simulink model "test_gFunction"  (R2018b)
settings: Solver=ode23  StartTime=0.0  StopTime=50*24*3600  RelTol=1e-3
values from neighbouring files (symbols this model uses):
  c4 = c41    [parameter_CARNOTews.m]
  gfunction = zeros(length(t_Trichter),length(r_Trichter))    [parameter_CARNOTews.m]
  L1 = 1/R1    [parameter_CARNOTews.m]
  lambdaErde = 2.0    (= 2)    [parameter_CARNOTews.m]
  Rechenradius = rm    (= 5)    [parameter_CARNOTews.m]
  T_null = TEarth0(end,:)'    [parameter_CARNOTews.m]
  t_start = 50*8560*3600    (= 1540800000)    [parameter_CARNOTews.m]
  Ts_Trichter = 7*24*3600    (= 604800)    [parameter_CARNOTews.m]
undefined symbols (not defined in the file or in its folder): dl
settings Model: SimulationMode=accelerator  Creator=drhf  LastModifiedBy=drhf

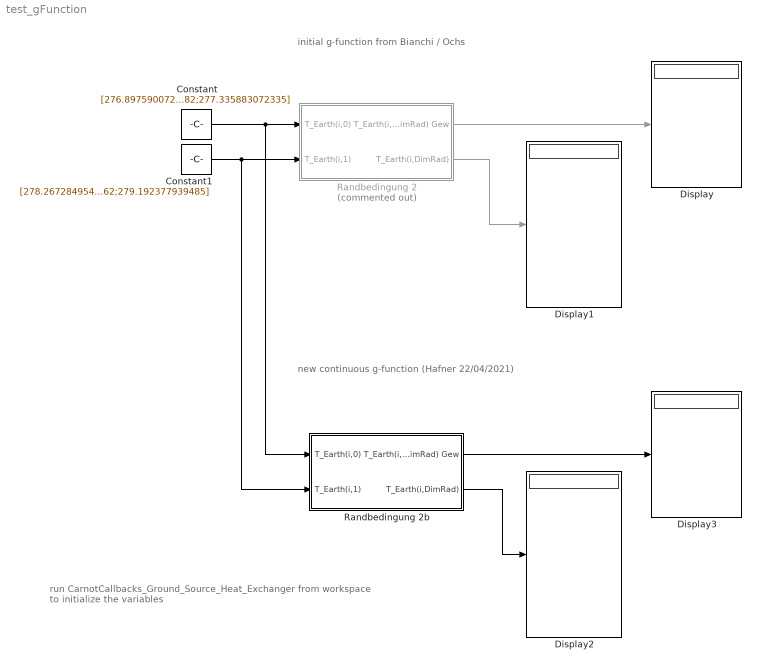
== system test_gFunction ==
  note: initial g-function from Bianchi / Ochs
  note: new continuous g-function (Hafner 22/04/2021)
  note: run CarnotCallbacks_Ground_Source_Heat_Exchanger
      | from workspace to initialize the variables
  Constant : Constant  Value=[276.897590072582;276.995261711216;277.100926067142;277.214495701082;277.335883072335]
  Constant1 : Constant  Value=[278.267284954817;278.488669745191;278.716706441616;278.951305488562;279.192377939485]
  Display{,1..3} (4 alike) : Display
  Randbedingung 2 : Subsystem  Commented=on
  Randbedingung 2b : Subsystem
  wires:
  Constant/1 -> Randbedingung 2b/1(T_Earth(i,0)), Randbedingung 2/1(T_Earth(i,0))
  Constant1/1 -> Randbedingung 2b/2(T_Earth(i,1)), Randbedingung 2/2(T_Earth(i,1))
  Randbedingung 2/1(T_Earth(i,DimRad) Gew) -> Display/1
  Randbedingung 2/2(T_Earth(i,DimRad)) -> Display1/1
  Randbedingung 2b/2(T_Earth(i,DimRad)) -> Display2/1
  Randbedingung 2b/1(T_Earth(i,DimRad) Gew) -> Display3/1

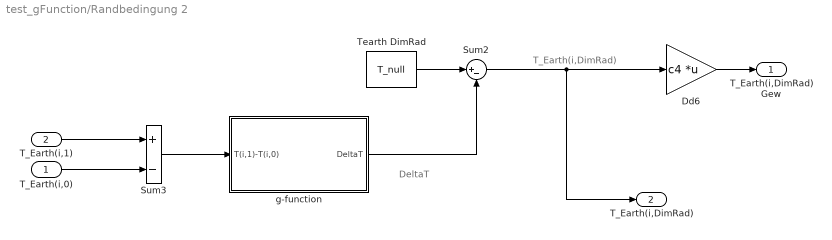
== system test_gFunction/Randbedingung 2 ==
  note: T_Earth(i,DimRad)
  note: DeltaT
  T_Earth(i,0) : Inport
  T_Earth(i,1) : Inport  Port=2
  Dd6 : Gain  Gain=c4  Multiplication=Matrix(K*u)  SaturateOnIntegerOverflow=on  OutDataTypeStr=Inherit: Same as input  ParamDataTypeStr=Inherit: Same as input
  Sum2 : Sum  Inputs=|+-  SaturateOnIntegerOverflow=on  InputSameDT=on  OutDataTypeStr=Inherit: Same as first input
  Sum3 : Sum  Inputs=+-  SaturateOnIntegerOverflow=on  InputSameDT=on  OutDataTypeStr=Inherit: Same as first input
  Tearth DimRad : Constant  Value=T_null  VectorParams1D=off
  g-function : Subsystem
  T_Earth(i,DimRad) Gew : Outport
  T_Earth(i,DimRad) : Outport  Port=2
  wires:
  Sum2/1 -> Dd6/1, T_Earth(i,DimRad)/1
  Tearth DimRad/1 -> Sum2/1
  T_Earth(i,1)/1 -> Sum3/1
  T_Earth(i,0)/1 -> Sum3/2
  Dd6/1 -> T_Earth(i,DimRad) Gew/1
  Sum3/1 -> g-function/1(T(i,1)-T(i,0))
  g-function/1(DeltaT) -> Sum2/2

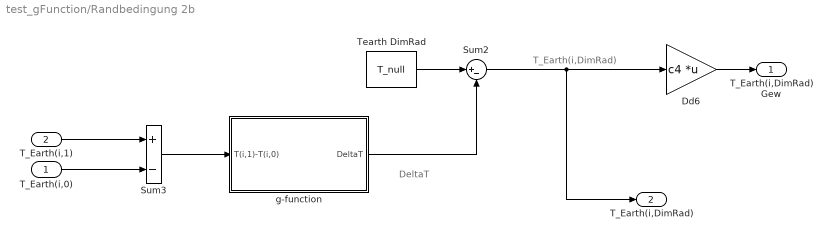
== system test_gFunction/Randbedingung 2b ==
  note: DeltaT
  note: T_Earth(i,DimRad)
  T_Earth(i,0) : Inport
  T_Earth(i,1) : Inport  Port=2
  Dd6 : Gain  Gain=c4  Multiplication=Matrix(K*u)  SaturateOnIntegerOverflow=on  OutDataTypeStr=Inherit: Same as input  ParamDataTypeStr=Inherit: Same as input
  Sum2 : Sum  Inputs=|+-  SaturateOnIntegerOverflow=on  InputSameDT=on  OutDataTypeStr=Inherit: Same as first input
  Sum3 : Sum  Inputs=+-  SaturateOnIntegerOverflow=on  InputSameDT=on  OutDataTypeStr=Inherit: Same as first input
  Tearth DimRad : Constant  Value=T_null  VectorParams1D=off
  g-function : Subsystem
  T_Earth(i,DimRad) Gew : Outport
  T_Earth(i,DimRad) : Outport  Port=2
  wires:
  g-function/1(DeltaT) -> Sum2/2
  Sum3/1 -> g-function/1(T(i,1)-T(i,0))
  Dd6/1 -> T_Earth(i,DimRad) Gew/1
  T_Earth(i,0)/1 -> Sum3/2
  T_Earth(i,1)/1 -> Sum3/1
  Tearth DimRad/1 -> Sum2/1
  Sum2/1 -> T_Earth(i,DimRad)/1, Dd6/1

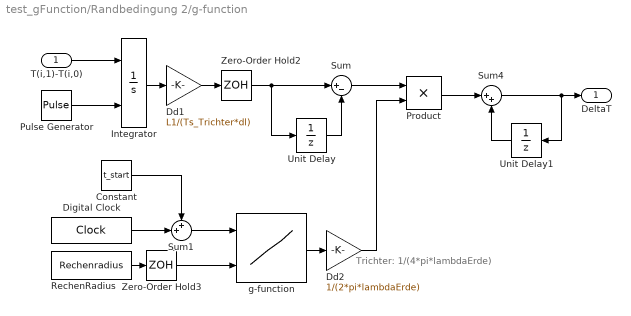
== system test_gFunction/Randbedingung 2/g-function ==
  note: Trichter: 1/(4*pi*lambdaErde)
  T(i,1)-T(i,0) : Inport
  Constant : Constant  Value=t_start
  Dd1 : Gain  Gain=L1/(Ts_Trichter*dl)  SaturateOnIntegerOverflow=on  OutDataTypeStr=Inherit: Same as input  ParamDataTypeStr=Inherit: Same as input
  Dd2 : Gain  Gain=1/(2*pi*lambdaErde)  SaturateOnIntegerOverflow=on  OutDataTypeStr=Inherit: Same as input  ParamDataTypeStr=Inherit: Same as input
  Digital Clock : DigitalClock
  Integrator : Integrator  ExternalReset=rising
  Product : Product  SaturateOnIntegerOverflow=on  RndMeth=Zero  InputSameDT=on  OutDataTypeStr=Inherit: Same as first input
  Pulse Generator : DiscretePulseGenerator  PulseType=Time based  Period=Ts_Trichter  PulseWidth=50  PhaseDelay=300
  RechenRadius : Constant  Value=Rechenradius  VectorParams1D=off
  Sum : Sum  Inputs=|+-  SaturateOnIntegerOverflow=on  InputSameDT=on  OutDataTypeStr=Inherit: Same as first input
  Sum1 : Sum  Inputs=++|  SaturateOnIntegerOverflow=on  InputSameDT=on  OutDataTypeStr=Inherit: Same as first input
  Sum4 : Sum  Inputs=|++  SaturateOnIntegerOverflow=on  InputSameDT=on  OutDataTypeStr=Inherit: Same as first input
  Unit Delay : UnitDelay
  Unit Delay1 : UnitDelay
  Zero-Order Hold2 : ZeroOrderHold
  Zero-Order Hold3 : ZeroOrderHold
  g-function : Lookup2D  RowIndex=t_Trichter  ColumnIndex=r_Trichter  Table=gfunction  SaturateOnIntegerOverflow=on  InputSameDT=on
  DeltaT : Outport
  wires:
  Constant/1 -> Sum1/1
  Sum1/1 -> g-function/1
  Digital Clock/1 -> Sum1/2
  Pulse Generator/1 -> Integrator/2
  Integrator/1 -> Dd1/1
  Dd1/1 -> Zero-Order Hold2/1
  Unit Delay/1 -> Sum/2
  Sum/1 -> Product/1
  g-function/1 -> Dd2/1
  RechenRadius/1 -> Zero-Order Hold3/1
  Product/1 -> Sum4/1
  Dd2/1 -> Product/2
  Unit Delay1/1 -> Sum4/2
  Sum4/1 -> Unit Delay1/1, DeltaT/1
  Zero-Order Hold3/1 -> g-function/2
  Zero-Order Hold2/1 -> Unit Delay/1, Sum/1
  T(i,1)-T(i,0)/1 -> Integrator/1

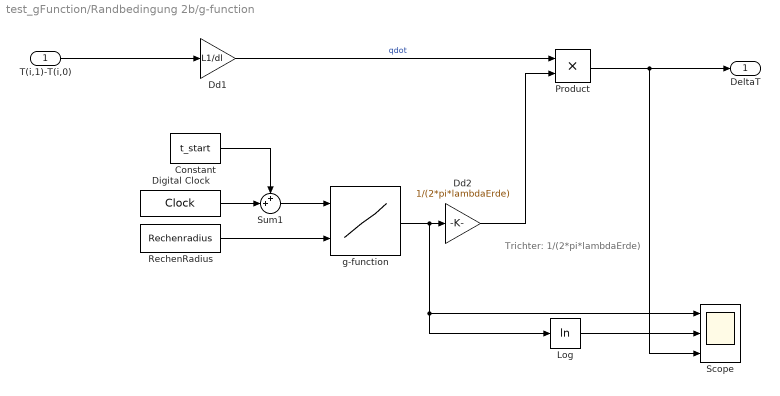
== system test_gFunction/Randbedingung 2b/g-function ==
  note: Trichter: 1/(2*pi*lambdaErde)
  T(i,1)-T(i,0) : Inport
  Constant : Constant  Value=t_start
  Dd1 : Gain  Gain=L1/dl  SaturateOnIntegerOverflow=on  OutDataTypeStr=Inherit: Same as input  ParamDataTypeStr=Inherit: Same as input
  Dd2 : Gain  Gain=1/(2*pi*lambdaErde)  SaturateOnIntegerOverflow=on  OutDataTypeStr=Inherit: Same as input  ParamDataTypeStr=Inherit: Same as input
  Digital Clock : DigitalClock
  Log : Math  Operator=log  SaturateOnIntegerOverflow=on
  Product : Product  SaturateOnIntegerOverflow=on  RndMeth=Zero  InputSameDT=on  OutDataTypeStr=Inherit: Same as first input
  RechenRadius : Constant  Value=Rechenradius  VectorParams1D=off
  Scope : Scope  NumInputPorts=3
  Sum1 : Sum  Inputs=++|  SaturateOnIntegerOverflow=on  InputSameDT=on  OutDataTypeStr=Inherit: Same as first input
  g-function : Lookup2D  RowIndex=t_Trichter  ColumnIndex=r_Trichter  Table=gfunction  SaturateOnIntegerOverflow=on  InputSameDT=on
  DeltaT : Outport
  wires:
  RechenRadius/1 -> g-function/2
  Dd2/1 -> Product/2
  Product/1 -> Scope/3, DeltaT/1
  g-function/1 -> Scope/1, Log/1, Dd2/1
  Dd1/1 -> Product/1  "qdot"
  T(i,1)-T(i,0)/1 -> Dd1/1
  Digital Clock/1 -> Sum1/2
  Constant/1 -> Sum1/1
  Sum1/1 -> g-function/1
  Log/1 -> Scope/2
